simulink model "RLFactory"  (R2021a)
settings: Solver=VariableStepAuto  StartTime=0.0  StopTime=1000  RelTol=1e-3
undefined symbols (not defined in the file): BLOCKEDTIMER, GOALSA, GOALSB, GOALSRL, INITAX, INITAY, INITBX, INITBY, MAXVELOA, MAXVELOB, SAFETYDISTANCEA, SAFETYDISTANCEB, THRESHOLDA, THRESHOLDB, TSA, TSB, TSRL
libraries: rllib x1
(part 2 of 2)

== system RLFactory/RLServiceRLRobot/RLServiceRLInfo/RLServiceCrashDetector/RLServiceEuclideanDistanceCalculator2 ==
  X : Inport
  Y : Inport  Port=2
  XOpp : Inport  Port=3
  YOpp : Inport  Port=4
  Square : Math  Operator=square  SaturateOnIntegerOverflow=on
  Square Root : Sqrt  SaturateOnIntegerOverflow=on
  Square1 : Math  Operator=square  SaturateOnIntegerOverflow=on
  Sum1 : Sum
  Sum3 : Sum  Inputs=+-
  Sum4 : Sum  Inputs=+-
  Dist : Outport
  wires:
  XOpp/1 -> Sum3/2
  X/1 -> Sum3/1
  Sum1/1 -> Square Root/1
  Sum4/1 -> Square1/1
  Square/1 -> Sum1/1
  Y/1 -> Sum4/1
  Square Root/1 -> Dist/1
  Square1/1 -> Sum1/2
  Sum3/1 -> Square/1
  YOpp/1 -> Sum4/2

== system RLFactory/RLServiceRLRobot/RLServiceRLInfo/RLServiceGoalTracker/RLServiceEuclideanDistanceCalculator ==
  X : Inport
  Y : Inport  Port=2
  GoalX : Inport  Port=3
  GoalY : Inport  Port=4
  Square : Math  Operator=square  SaturateOnIntegerOverflow=on
  Square Root : Sqrt  SaturateOnIntegerOverflow=on
  Square1 : Math  Operator=square  SaturateOnIntegerOverflow=on
  Sum1 : Sum
  Sum3 : Sum  Inputs=+-
  Sum4 : Sum  Inputs=+-
  DistGoal : Outport
  wires:
  GoalX/1 -> Sum3/2
  X/1 -> Sum3/1
  Sum1/1 -> Square Root/1
  Sum4/1 -> Square1/1
  Square/1 -> Sum1/1
  Y/1 -> Sum4/1
  Square Root/1 -> DistGoal/1
  Square1/1 -> Sum1/2
  Sum3/1 -> Square/1
  GoalY/1 -> Sum4/2

== system RLFactory/RLServiceRLRobot/RLServiceRLRobotSensor/RLServiceARobotSensorSubsystem/RLServiceDirectionCalculator ==
  OppX : Inport
  OppY : Inport  Port=2
  Demux : Demux  Outputs=2
  Mux : Mux  Inputs=2
  Sign : Signum
  Sign1 : Signum
  Sum : Sum  Inputs=+-
  Unit Delay : UnitDelay  SampleTime=TSRL  HasFrameUpgradeWarning=on
  DirOppX : Outport
  DirOppY : Outport  Port=2
  wires:
  Mux/1 -> Unit Delay/1, Sum/1
  Unit Delay/1 -> Sum/2
  Sum/1 -> Demux/1
  Demux/1 -> Sign1/1
  Demux/2 -> Sign/1
  Sign1/1 -> DirOppX/1
  Sign/1 -> DirOppY/1
  OppX/1 -> Mux/1
  OppY/1 -> Mux/2

== system RLFactory/RLServiceRLRobot/RLServiceRLRobotSensor/RLServiceBRobotSensorSubsystem/RLServiceDirectionCalculator ==
  OppX : Inport
  OppY : Inport  Port=2
  Demux : Demux  Outputs=2
  Mux : Mux  Inputs=2
  Sign : Signum
  Sign1 : Signum
  Sum : Sum  Inputs=+-
  Unit Delay : UnitDelay  SampleTime=TSRL  HasFrameUpgradeWarning=on
  DirOppX : Outport
  DirOppY : Outport  Port=2
  wires:
  Mux/1 -> Unit Delay/1, Sum/1
  Unit Delay/1 -> Sum/2
  Sum/1 -> Demux/1
  Demux/1 -> Sign1/1
  Demux/2 -> Sign/1
  Sign1/1 -> DirOppX/1
  Sign/1 -> DirOppY/1
  OppX/1 -> Mux/1
  OppY/1 -> Mux/2
